simulink subsystem "EPS_Physical_Model"  (R2024a)
settings: Solver=VariableStepAuto  StartTime=0.0  StopTime=10.0  RelTol=1e-3
undefined symbols (not defined in the file): dcVoltage, Power, satellite, sensor
libraries: nesl_utility x25, fl_lib x24, ee_lib x6, autolibdatasheetbattery x1
(part 2 of 2)

== system EPS_Physical_Model/Solar Panels1/Solar Panel +Y/Solar Panel1 ==
  Current-Controlled Current Source : fl_lib/Electrical/Electrical Sources/Current-Controlled Current Source  K=-1  i1_specify=off  i1_priority=None  i1=0 A  i1_nominal_specify=off  i1_nominal_value=1  i1_nominal_unit=A  i2_specify=off  i2_priority=None  i2=0 A  i2_nominal_specify=off  i2_nominal_value=1  i2_nominal_unit=A
      settings: InternalSimscapePortConfiguration="{\"Bottom\":[],\"Left\":[{\"id\":\"p1\",\"label\":\"+\",\"type\":\"foundation.electrical.electrical\"},{\"id\":\"head\",\"label\":\"\",\"type\":\"foundation.electrical.electrical\"}],\"Right\":[{\"id\":\"n1\",\"label\":\"-\",\"type\":\"foundation.electrical.electrical\"},{\"id\":\"tail\",\"label\":\"\",\"type\":\"foundation.electrical.electrical\"}],\"Top\":[]}"
  Solar Cell : ee_lib/Sources/Solar Cell  PartSpecification="{\"DatasetId\":\"AzurSpace|3C44_30sqmm|simscape.electrical.solarCell\",\"DisplayName\":\"AzurSpace:3C44_30sqmm\"}"  prm=3  Isc=1.19 % Datasheet derived A  Voc=3.08 % Datasheet derived V  Is=2.73592960844769e-35 % Datasheet derived A  Is2=1.16779785679844e-37 % Datasheet derived A  Iph=1.19000472592367 % Datasheet derived A  Ir0=250000 % Datasheet derived W/m^2  ec=1.50303550965723 % Datasheet derived  N2=1.59525933684062 % Datasheet derived  Rs=0.104281524604326 % Datasheet derived Ohm  Rp=26248.1045129446 % Datasheet derived Ohm  N_series=1 % Datasheet derived  N_parallel=1 % Datasheet derived  TIPH1=0.000799987520460482 % Datasheet derived 1/K  EG=1.441 % Datasheet derived eV  TXIS1=92.8777524632801 % Datasheet derived  TXIS2=227.92622072394 % Datasheet derived  TRS1=0.0216421647602992 % Datasheet derived  TRP1=0 % Parameter not set  Tmeas=25 % Datasheet derived degC  TFIXED=25 % Datasheet derived degC  thermal_mass=100 % Parameter not set J/K  initial_temperature=25 degC
      settings: AttributesFormatString=AzurSpace:3C44_30sqmm
  Solar Cell1 : ee_lib/Sources/Solar Cell  PartSpecification="{\"DatasetId\":\"AzurSpace|3C44_30sqmm|simscape.electrical.solarCell\",\"DisplayName\":\"AzurSpace:3C44_30sqmm\"}"  prm=3  Isc=1.19 % Datasheet derived A  Voc=3.08 % Datasheet derived V  Is=2.73592960844769e-35 % Datasheet derived A  Is2=1.16779785679844e-37 % Datasheet derived A  Iph=1.19000472592367 % Datasheet derived A  Ir0=250000 % Datasheet derived W/m^2  ec=1.50303550965723 % Datasheet derived  N2=1.59525933684062 % Datasheet derived  Rs=0.104281524604326 % Datasheet derived Ohm  Rp=26248.1045129446 % Datasheet derived Ohm  N_series=1 % Datasheet derived  N_parallel=1 % Datasheet derived  TIPH1=0.000799987520460482 % Datasheet derived 1/K  EG=1.441 % Datasheet derived eV  TXIS1=92.8777524632801 % Datasheet derived  TXIS2=227.92622072394 % Datasheet derived  TRS1=0.0216421647602992 % Datasheet derived  TRP1=0 % Parameter not set  Tmeas=25 % Datasheet derived degC  TFIXED=25 % Datasheet derived degC  thermal_mass=100 % Parameter not set J/K  initial_temperature=25 degC
      settings: AttributesFormatString=AzurSpace:3C44_30sqmm
  Ir : PMIOPort  Side=Left
  + : PMIOPort  Port=2  Side=Right
  - : PMIOPort  Port=3  Side=Right
  connections:
  Current-Controlled Current Source/LConn2 -- -/RConn1 -- Solar Cell/RConn1
  Ir/RConn1 -- Solar Cell/LConn1
  Current-Controlled Current Source/LConn1 -- Solar Cell/LConn2
  Current-Controlled Current Source/RConn1 -- Current-Controlled Current Source/RConn2 -- +/RConn1

== system EPS_Physical_Model/Solar Panels1/Solar Panel -X/Solar Panel2 ==
  Current-Controlled Current Source : fl_lib/Electrical/Electrical Sources/Current-Controlled Current Source  K=-1  i1_specify=off  i1_priority=None  i1=0 A  i1_nominal_specify=off  i1_nominal_value=1  i1_nominal_unit=A  i2_specify=off  i2_priority=None  i2=0 A  i2_nominal_specify=off  i2_nominal_value=1  i2_nominal_unit=A
      settings: InternalSimscapePortConfiguration="{\"Bottom\":[],\"Left\":[{\"id\":\"p1\",\"label\":\"+\",\"type\":\"foundation.electrical.electrical\"},{\"id\":\"head\",\"label\":\"\",\"type\":\"foundation.electrical.electrical\"}],\"Right\":[{\"id\":\"n1\",\"label\":\"-\",\"type\":\"foundation.electrical.electrical\"},{\"id\":\"tail\",\"label\":\"\",\"type\":\"foundation.electrical.electrical\"}],\"Top\":[]}"
  Solar Cell : ee_lib/Sources/Solar Cell  PartSpecification="{\"DatasetId\":\"AzurSpace|3C44_30sqmm|simscape.electrical.solarCell\",\"DisplayName\":\"AzurSpace:3C44_30sqmm\"}"  prm=3  Isc=1.19 % Datasheet derived A  Voc=3.08 % Datasheet derived V  Is=2.73592960844769e-35 % Datasheet derived A  Is2=1.16779785679844e-37 % Datasheet derived A  Iph=1.19000472592367 % Datasheet derived A  Ir0=250000 % Datasheet derived W/m^2  ec=1.50303550965723 % Datasheet derived  N2=1.59525933684062 % Datasheet derived  Rs=0.104281524604326 % Datasheet derived Ohm  Rp=26248.1045129446 % Datasheet derived Ohm  N_series=1 % Datasheet derived  N_parallel=1 % Datasheet derived  TIPH1=0.000799987520460482 % Datasheet derived 1/K  EG=1.441 % Datasheet derived eV  TXIS1=92.8777524632801 % Datasheet derived  TXIS2=227.92622072394 % Datasheet derived  TRS1=0.0216421647602992 % Datasheet derived  TRP1=0 % Parameter not set  Tmeas=25 % Datasheet derived degC  TFIXED=25 % Datasheet derived degC  thermal_mass=100 % Parameter not set J/K  initial_temperature=25 degC
      settings: AttributesFormatString=AzurSpace:3C44_30sqmm
  Ir : PMIOPort  Side=Left
  + : PMIOPort  Port=2  Side=Right
  - : PMIOPort  Port=3  Side=Right
  connections:
  Current-Controlled Current Source/LConn2 -- -/RConn1 -- Solar Cell/RConn1
  Ir/RConn1 -- Solar Cell/LConn1
  Current-Controlled Current Source/LConn1 -- Solar Cell/LConn2
  Current-Controlled Current Source/RConn1 -- Current-Controlled Current Source/RConn2 -- +/RConn1

== system EPS_Physical_Model/Solar Panels1/Solar Panel -Y/Solar Panel1 ==
  Current-Controlled Current Source : fl_lib/Electrical/Electrical Sources/Current-Controlled Current Source  K=-1  i1_specify=off  i1_priority=High  i1=0.01 A  i1_nominal_specify=off  i1_nominal_value=1  i1_nominal_unit=A  i2_specify=off  i2_priority=None  i2=0 A  i2_nominal_specify=off  i2_nominal_value=1  i2_nominal_unit=A
      settings: InternalSimscapePortConfiguration="{\"Bottom\":[],\"Left\":[{\"id\":\"p1\",\"label\":\"+\",\"type\":\"foundation.electrical.electrical\"},{\"id\":\"head\",\"label\":\"\",\"type\":\"foundation.electrical.electrical\"}],\"Right\":[{\"id\":\"n1\",\"label\":\"-\",\"type\":\"foundation.electrical.electrical\"},{\"id\":\"tail\",\"label\":\"\",\"type\":\"foundation.electrical.electrical\"}],\"Top\":[]}"
  Solar Cell : ee_lib/Sources/Solar Cell  PartSpecification="{\"DatasetId\":\"AzurSpace|3C44_30sqmm|simscape.electrical.solarCell\",\"DisplayName\":\"AzurSpace:3C44_30sqmm\"}"  prm=3  Isc=1.19 % Datasheet derived A  Voc=3.08 % Datasheet derived V  Is=2.73592960844769e-35 % Datasheet derived A  Is2=1.16779785679844e-37 % Datasheet derived A  Iph=1.19000472592367 % Datasheet derived A  Ir0=250000 % Datasheet derived W/m^2  ec=1.50303550965723 % Datasheet derived  N2=1.59525933684062 % Datasheet derived  Rs=0.104281524604326 % Datasheet derived Ohm  Rp=26248.1045129446 % Datasheet derived Ohm  N_series=1 % Datasheet derived  N_parallel=1 % Datasheet derived  TIPH1=0.000799987520460482 % Datasheet derived 1/K  EG=1.441 % Datasheet derived eV  TXIS1=92.8777524632801 % Datasheet derived  TXIS2=227.92622072394 % Datasheet derived  TRS1=0.0216421647602992 % Datasheet derived  TRP1=0 % Parameter not set  Tmeas=25 % Datasheet derived degC  TFIXED=25 % Datasheet derived degC  thermal_mass=100 % Parameter not set J/K  initial_temperature=25 degC
      settings: AttributesFormatString=AzurSpace:3C44_30sqmm
  Ir : PMIOPort  Side=Left
  + : PMIOPort  Port=2  Side=Right
  - : PMIOPort  Port=3  Side=Right
  connections:
  Current-Controlled Current Source/LConn2 -- -/RConn1 -- Solar Cell/RConn1
  Ir/RConn1 -- Solar Cell/LConn1
  Current-Controlled Current Source/LConn1 -- Solar Cell/LConn2
  Current-Controlled Current Source/RConn1 -- Current-Controlled Current Source/RConn2 -- +/RConn1

== system EPS_Physical_Model/Solar Panels1/Solar Panel Z/Solar Panel1 ==
  Current-Controlled Current Source : fl_lib/Electrical/Electrical Sources/Current-Controlled Current Source  K=-1  i1_specify=off  i1_priority=None  i1=0 A  i1_nominal_specify=off  i1_nominal_value=1  i1_nominal_unit=A  i2_specify=off  i2_priority=None  i2=0 A  i2_nominal_specify=off  i2_nominal_value=1  i2_nominal_unit=A
      settings: InternalSimscapePortConfiguration="{\"Bottom\":[],\"Left\":[{\"id\":\"p1\",\"label\":\"+\",\"type\":\"foundation.electrical.electrical\"},{\"id\":\"head\",\"label\":\"\",\"type\":\"foundation.electrical.electrical\"}],\"Right\":[{\"id\":\"n1\",\"label\":\"-\",\"type\":\"foundation.electrical.electrical\"},{\"id\":\"tail\",\"label\":\"\",\"type\":\"foundation.electrical.electrical\"}],\"Top\":[]}"
  Solar Cell : ee_lib/Sources/Solar Cell  PartSpecification="{\"DatasetId\":\"AzurSpace|3C44_30sqmm|simscape.electrical.solarCell\",\"DisplayName\":\"AzurSpace:3C44_30sqmm\"}"  prm=3  Isc=1.19 % Datasheet derived A  Voc=3.08 % Datasheet derived V  Is=2.73592960844769e-35 % Datasheet derived A  Is2=1.16779785679844e-37 % Datasheet derived A  Iph=1.19000472592367 % Datasheet derived A  Ir0=250000 % Datasheet derived W/m^2  ec=1.50303550965723 % Datasheet derived  N2=1.59525933684062 % Datasheet derived  Rs=0.104281524604326 % Datasheet derived Ohm  Rp=26248.1045129446 % Datasheet derived Ohm  N_series=1 % Datasheet derived  N_parallel=1 % Datasheet derived  TIPH1=0.000799987520460482 % Datasheet derived 1/K  EG=1.441 % Datasheet derived eV  TXIS1=92.8777524632801 % Datasheet derived  TXIS2=227.92622072394 % Datasheet derived  TRS1=0.0216421647602992 % Datasheet derived  TRP1=0 % Parameter not set  Tmeas=25 % Datasheet derived degC  TFIXED=25 % Datasheet derived degC  thermal_mass=100 % Parameter not set J/K  initial_temperature=25 degC
      settings: AttributesFormatString=AzurSpace:3C44_30sqmm
  Ir : PMIOPort  Side=Left
  + : PMIOPort  Port=2  Side=Right
  - : PMIOPort  Port=3  Side=Right
  connections:
  Current-Controlled Current Source/LConn2 -- -/RConn1 -- Solar Cell/RConn1
  Ir/RConn1 -- Solar Cell/LConn1
  Current-Controlled Current Source/LConn1 -- Solar Cell/LConn2
  Current-Controlled Current Source/RConn1 -- Current-Controlled Current Source/RConn2 -- +/RConn1

== system EPS_Physical_Model/PCDU Board Model/BatteryChargerRegulators/MPPT 1/AC Current Sensor2 ==
  Current Sensor : fl_lib/Electrical/Electrical Sensors/Current Sensor
  PS-Simulink Converter : nesl_utility/PS-Simulink Converter  PhysicalDomain=network_engine_domain  SubClassName=ps_output  LeftPortType=input  RightPortType=output  PseudoPeriodic=off  Frequencies=[]  VectorFormat=1-D array  Unit=1  AffineConversion=off
  Sensor dynamics : TransferFcn  Numerator=1  Denominator=[1/sensor.samplingFreq 1]
  - : PMIOPort  Side=Left
  + : PMIOPort  Port=2  Side=Right
  tag scope: Imppt_x=global
  wires:
  PS-Simulink Converter/1 -> Sensor dynamics/1
  Sensor dynamics/1 -> [Imppt_x]
  connections:
  Current Sensor/RConn1 -- PS-Simulink Converter/LConn1
  +/RConn1 -- Current Sensor/LConn1
  Current Sensor/RConn2 -- -/RConn1

== system EPS_Physical_Model/PCDU Board Model/BatteryChargerRegulators/MPPT 1/DC Current Sensor ==
  Current Sensor : fl_lib/Electrical/Electrical Sensors/Current Sensor
      settings: LogSimulationData=on
  PS-Simulink Converter : nesl_utility/PS-Simulink Converter  PhysicalDomain=network_engine_domain  SubClassName=ps_output  LeftPortType=input  RightPortType=output  PseudoPeriodic=off  Frequencies=[]  VectorFormat=1-D array  Unit=1  AffineConversion=off
  Sensor dynamics : TransferFcn  Numerator=1  Denominator=[1/sensor.samplingFreq 1]
  - : PMIOPort  Side=Left
  + : PMIOPort  Port=2  Side=Right
  tag scope: Icell_x=global
  wires:
  PS-Simulink Converter/1 -> Sensor dynamics/1
  Sensor dynamics/1 -> [Icell_x]
  connections:
  Current Sensor/RConn2 -- -/RConn1
  +/RConn1 -- Current Sensor/LConn1
  Current Sensor/RConn1 -- PS-Simulink Converter/LConn1

== system EPS_Physical_Model/PCDU Board Model/BatteryChargerRegulators/MPPT 1/DC Output Voltage Sensor ==
  PS-Simulink Converter : nesl_utility/PS-Simulink Converter  PhysicalDomain=network_engine_domain  SubClassName=ps_output  LeftPortType=input  RightPortType=output  PseudoPeriodic=off  Frequencies=[]  VectorFormat=1-D array  Unit=1  AffineConversion=off
  Sensor dynamics : TransferFcn  Numerator=1  Denominator=[1/sensor.samplingFreq 1]
  Voltage Sensor : fl_lib/Electrical/Electrical Sensors/Voltage Sensor
  - : PMIOPort  Side=Left
  + : PMIOPort  Port=2  Side=Right
  tag scope: Vmppt_x=global
  wires:
  PS-Simulink Converter/1 -> Sensor dynamics/1
  Sensor dynamics/1 -> [Vmppt_x]
  connections:
  Voltage Sensor/RConn2 -- -/RConn1
  Voltage Sensor/RConn1 -- PS-Simulink Converter/LConn1
  Voltage Sensor/LConn1 -- +/RConn1

== system EPS_Physical_Model/PCDU Board Model/BatteryChargerRegulators/MPPT 1/DC Voltage Sensor ==
  PS-Simulink Converter : nesl_utility/PS-Simulink Converter  PhysicalDomain=network_engine_domain  SubClassName=ps_output  LeftPortType=input  RightPortType=output  PseudoPeriodic=off  Frequencies=[]  VectorFormat=1-D array  Unit=1  AffineConversion=off
  Sensor dynamics : TransferFcn  Numerator=1  Denominator=[1/sensor.samplingFreq 1]
  Voltage Sensor : fl_lib/Electrical/Electrical Sensors/Voltage Sensor
      settings: LogSimulationData=on
  - : PMIOPort  Side=Left
  + : PMIOPort  Port=2  Side=Right
  tag scope: Vcell_x=global
  wires:
  PS-Simulink Converter/1 -> Sensor dynamics/1
  Sensor dynamics/1 -> [Vcell_x]
  connections:
  Voltage Sensor/LConn1 -- +/RConn1
  Voltage Sensor/RConn1 -- PS-Simulink Converter/LConn1
  Voltage Sensor/RConn2 -- -/RConn1

== system EPS_Physical_Model/PCDU Board Model/BatteryChargerRegulators/MPPT 1/Load ==
  " " : Constant
  " (Average DC Voltage)^2" : Constant  Value=dcVoltage.avgDCVoltage*dcVoltage.avgDCVoltage
  " 1" : Constant  Value=1.5
  Load Power (kW) : Gain  Gain=1.688857025146485
  Simulink-PS Converter1 : nesl_utility/Simulink-PS Converter  PhysicalDomain=network_engine_domain  SubClassName=ps_input  LeftPortType=input  RightPortType=output  PseudoPeriodic=off  Frequencies=[]  NoiseDistribution=none  NoiseParameters=[]  Unit=1  AffineConversion=off  FilteringAndDerivatives=provide  SimscapeFilterOrder=1  InputFilterTimeConstant=0.001  UdotUserProvided=0
  Switch : Switch  Criteria=u2 > Threshold  SaturateOnIntegerOverflow=off  InputSameDT=off
  V^2/P : Product  Inputs=*/
  kW2W : Gain  Gain=1000
  R : PMIOPort  Side=Right
  wires:
  " "/1 -> Load Power (kW)/1
  Load Power (kW)/1 -> Switch/1, Switch/2
  " 1"/1 -> Switch/3
  " (Average DC Voltage)^2"/1 -> V^2/P/1
  V^2/P/1 -> Simulink-PS Converter1/1
  Switch/1 -> kW2W/1
  kW2W/1 -> V^2/P/2
  connections:
  Simulink-PS Converter1/RConn1 -- R/RConn1

== system EPS_Physical_Model/PCDU Board Model/BatteryChargerRegulators/MPPT 1/MPPT ==
  Bus Selector : BusSelector  OutputSignals=signal1
  SEPIC converter : Subsystem
  Switch1 : Switch  SaturateOnIntegerOverflow=off  InputSameDT=off
  in + : PMIOPort  Side=Left
  in - : PMIOPort  Port=2  Side=Left
  out + : PMIOPort  Port=3  Side=Right
  out - : PMIOPort  Port=4  Side=Right
  wires:
  [control_comm] -> Bus Selector/1

== system EPS_Physical_Model/PCDU Board Model/BatteryChargerRegulators/MPPT 2/EMI Filters ==
  In1 : Inport
  Solar X : Outport
  wires:
  In1/1 -> Solar X/1

== system EPS_Physical_Model/PCDU Board Model/BatteryChargerRegulators/MPPT 2/I & V Measurment ==
  Solar X : Inport
  V solar : Outport
  wires:
  Solar X/1 -> V solar/1

== system EPS_Physical_Model/PCDU Board Model/BatteryChargerRegulators/MPPT 2/I & V Measurment1 ==
  In1 : Inport
  V solar : Outport
  wires:
  In1/1 -> V solar/1

== system EPS_Physical_Model/PCDU Board Model/BatteryChargerRegulators/MPPT 2/MPPT ==
  In1 : Inport
  SEPIC converter : Subsystem
  Out1 : Outport
  wires:
  SEPIC converter/1(Out1) -> Out1/1
  In1/1 -> SEPIC converter/1(In1)

== system EPS_Physical_Model/PCDU Board Model/BatteryChargerRegulators/MPPT 3/EMI Filters ==
  In1 : Inport
  Solar X : Outport
  wires:
  In1/1 -> Solar X/1

== system EPS_Physical_Model/PCDU Board Model/BatteryChargerRegulators/MPPT 3/I & V Measurment ==
  Solar X : Inport
  V solar : Outport
  wires:
  Solar X/1 -> V solar/1

== system EPS_Physical_Model/PCDU Board Model/BatteryChargerRegulators/MPPT 3/I & V Measurment1 ==
  In1 : Inport
  V solar : Outport
  wires:
  In1/1 -> V solar/1

== system EPS_Physical_Model/PCDU Board Model/BatteryChargerRegulators/MPPT 3/MPPT ==
  In1 : Inport
  SEPIC converter : Subsystem
  Out1 : Outport
  wires:
  SEPIC converter/1(Out1) -> Out1/1
  In1/1 -> SEPIC converter/1(In1)

== system EPS_Physical_Model/PCDU Board Model/BatteryChargerRegulators/MPPT 1/MPPT/SEPIC converter ==
  In1 : Inport
  Out1 : Outport
  wires:
  In1/1 -> Out1/1

== system EPS_Physical_Model/PCDU Board Model/BatteryChargerRegulators/MPPT 2/MPPT/SEPIC converter ==
  In1 : Inport
  Out1 : Outport
  wires:
  In1/1 -> Out1/1

== system EPS_Physical_Model/PCDU Board Model/BatteryChargerRegulators/MPPT 3/MPPT/SEPIC converter ==
  In1 : Inport
  Out1 : Outport
  wires:
  In1/1 -> Out1/1
